simulink model "Simu_2"  (R2024a)
settings: Solver=VariableStepAuto  StartTime=0.0  StopTime=10  FixedStep=1e-4  RelTol=1e-3
undefined symbols (not defined in the file): B, K, kd, ki, kp, M, T
libraries: dspsrcs4 x2, slpidlib x1
settings Model: Creator=a2152355  LastModifiedBy=a2152355

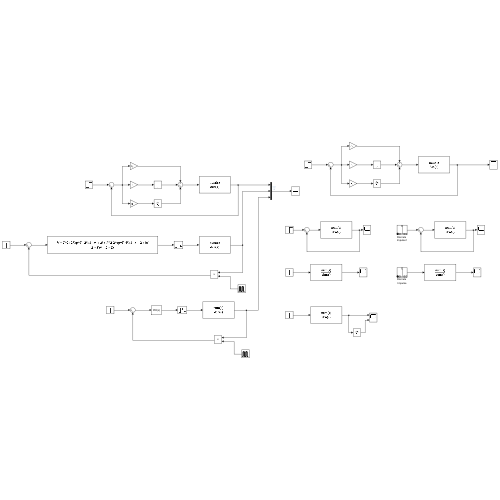
[thumbnail: Simulink's stored preview of the top-level diagram]
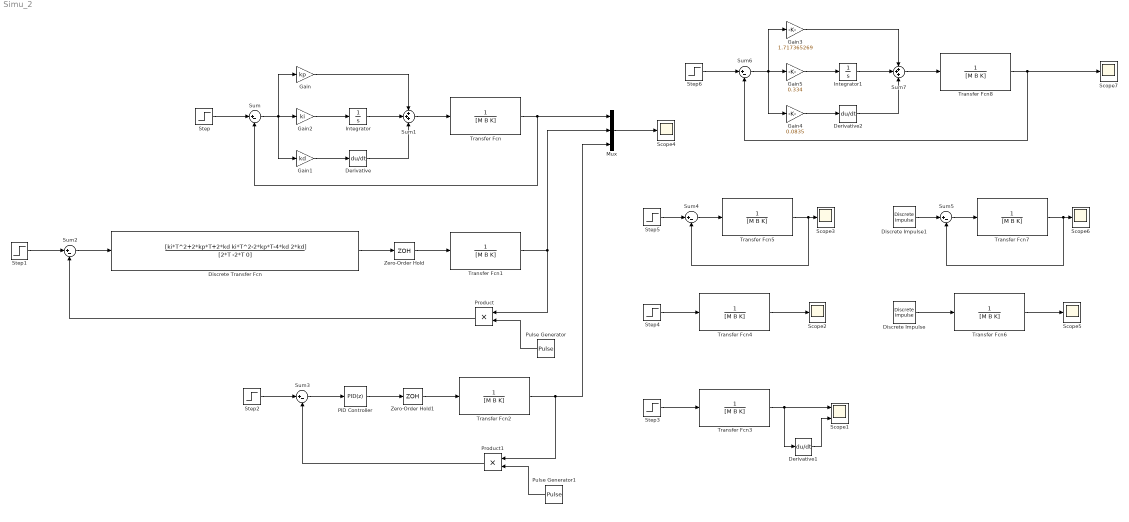
== system Simu_2 ==
  Derivative : Derivative
  Derivative1 : Derivative
  Derivative2 : Derivative
  Discrete Transfer Fcn : DiscreteTransferFcn  Numerator=[ki*T^2+2*kp*T+2*kd ki*T^2-2*kp*T-4*kd 2*kd]  Denominator=[2*T -2*T 0]
  Discrete Impulse : dspsrcs4/Discrete  Impulse  Delay=0  SampleTime=1  FrameSample=1  OutputFrames=off  dataType=double  isSigned=on  wordLen=16  udDataType=sfix(16)  fracBitsMode=Best precision  numFracBits=15  OutDataTypeStr=double  LastOutDataTypeStr=double
  Discrete Impulse1 : dspsrcs4/Discrete  Impulse  Delay=0  SampleTime=1  FrameSample=1  OutputFrames=off  dataType=double  isSigned=on  wordLen=16  udDataType=sfix(16)  fracBitsMode=Best precision  numFracBits=15  OutDataTypeStr=double  LastOutDataTypeStr=double
  Gain : Gain  Gain=kp
  Gain1 : Gain  Gain=kd
  Gain2 : Gain  Gain=ki
  Gain3 : Gain  Gain=1.717365269
  Gain4 : Gain  Gain=0.0835
  Gain5 : Gain  Gain=0.334
  Integrator : Integrator
  Integrator1 : Integrator
  Mux : Mux  Inputs=3
  PID Controller : slpidlib/PID Controller  Controller=PID  Form=Parallel  TimeDomain=Discrete-time  UseExternalTs=off  SampleTime=T  IntegratorMethod=Forward Euler  FilterMethod=Forward Euler  ControllerParametersSource=internal  P=kp  I=ki  UseKiTs=off  D=kd  UseExternalDerivativeSource=off  N=100  UseFilter=on  TunerSelectOption=Transfer Function Based (PID Tuner App)  InitialConditionSource=internal  InitialConditionForIntegrator=0  InitialConditionForFilter=0  DifferentiatorICPrevScaledInput=0  ExternalReset=none  TrackingMode=off  Kt=1  LimitOutput=off  SatLimitsSource=internal  UpperSaturationLimit=inf  LowerSaturationLimit=-inf  LinearizeAsGain=on  AntiWindupMode=none  Kb=1  LimitIntegrator=off  UpperIntegratorSaturationLimit=inf  LowerIntegratorSaturationLimit=-inf  POutMin=[]  POutMax=[]  IOutMin=[]  IOutMax=[]  DOutMin=[]  DOutMax=[]  NOutMin=[]  NOutMax=[]  SumOutMin=[]  SumOutMax=[]  SaturationOutMin=[]  SaturationOutMax=[]  PParamMin=[]  PParamMax=[]  IParamMin=[]  IParamMax=[]  DParamMin=[]  DParamMax=[]  NParamMin=[]  NParamMax=[]  KbParamMin=[]  KbParamMax=[]  KtParamMin=[]  KtParamMax=[]  KbOutMin=[]  KbOutMax=[]  KtOutMin=[]  KtOutMax=[]  IntegratorOutMin=[]  IntegratorOutMax=[]  FilterOutMin=[]  FilterOutMax=[]  SumI1OutMin=[]  SumI1OutMax=[]  SumI2OutMin=[]  SumI2OutMax=[]  SumI3OutMin=[]  SumI3OutMax=[]  SumI4OutMin=[]  SumI4OutMax=[]  SumDOutMin=[]  SumDOutMax=[]  DifferentiatorOutMin=[]  DifferentiatorOutMax=[]  FilterDiffOutCoefMin=[]  FilterDiffOutCoefMax=[]  ReciprocalOutMin=[]  ReciprocalOutMax=[]  SumDenOutMin=[]  SumDenOutMax=[]  SumNumOutMin=[]  SumNumOutMax=[]  DivideOutMin=[]  DivideOutMax=[]  UdiffTsProdOutMin=[]  UdiffTsProdOutMax=[]  NTsProdOutMin=[]  NTsProdOutMax=[]  UintegralTsProdOutMin=[]  UintegralTsProdOutMax=[]  UngainTsProdOutMin=[]  UngainTsProdOutMax=[]  ClampingZeroOutDataTypeStr=Inherit: Inherit via back propagation  ClampingZeroOutMin=[]  ClampingZeroOutMax=[]  FilterDenConstantOutDataTypeStr=Inherit: Inherit via back propagation  FilterDenConstantOutMin=[]  FilterDenConstantOutMax=[]  PCopyOutDataTypeStr=Inherit: Inherit via back propagation  PCopyOutMin=[]  PCopyOutMax=[]  NCopyOutDataTypeStr=Inherit: Inherit via back propagation  NCopyOutMin=[]  NCopyOutMax=[]  IntegratorContinuousStateAttributes=''  IntegratorStateMustResolveToSignalObject=off  IntegratorRTWStateStorageClass=Auto  FilterContinuousStateAttributes=''  FilterStateMustResolveToSignalObject=off  FilterRTWStateStorageClass=Auto  ParallelPVariant=InternalParameters  IdealPVariant=Disabled  IVariant=InternalParameters  DVariant=InternalParameters  IntegratorVariant=Discrete  SatVariant=Disabled  AWVariant=Passthrough  PCopyVariant=Disabled  TRVariant=Disabled  FdbkBlocksVariant=Forward  IdealPFdbkVariant=Disabled  SatFdbkVariant=Disabled  DerivativeFilterVariant=ForwardEulerFilter  NVariant=InternalParameters  NCopyVariant=Disabled  FilterICVariant=InternalICsFilter  IntegratorICVariant=InternalICs  ExternalResetVariant=Disabled  TRSumVariant=Passthrough  SumFdbkVariant=Disabled  SumVariant=Sum_PID  TsampFilterVariant=InternalTs  TsampNgainVariant=Passthrough  TsampIntegralVariant=Disabled_SignalSpec  ExternalSaturationOutDataTypeStr=Inherit: Same as second input  DerivativeSourceVariant=ErrorSignal
  Product : Product
  Product1 : Product
  Pulse Generator : DiscretePulseGenerator  PulseType=Time based  Period=T  PulseWidth=0.1
  Pulse Generator1 : DiscretePulseGenerator  PulseType=Time based  Period=T  PulseWidth=0.1
  Scope1 : Scope  NumInputPorts=2
  Scope{2..7} (6 alike) : Scope
  Step{,1..6} (7 alike) : Step  SampleTime=0
  Sum{,2..6} (6 alike) : Sum  Inputs=|+-
  Sum1 : Sum  Inputs=+++
  Sum7 : Sum  Inputs=+++
  Transfer Fcn{,1..8} (9 alike) : TransferFcn  Denominator=[M B K]
  Zero-Order Hold : ZeroOrderHold  SampleTime=T
  Zero-Order Hold1 : ZeroOrderHold  SampleTime=T
  wires:
  Transfer Fcn/1 -> Mux/1, Sum/2
  Sum/1 -> Gain2/1, Gain/1, Gain1/1
  Step/1 -> Sum/1
  Gain1/1 -> Derivative/1
  Derivative/1 -> Sum1/3
  Integrator/1 -> Sum1/2
  Gain/1 -> Sum1/1
  Gain2/1 -> Integrator/1
  Sum1/1 -> Transfer Fcn/1
  Transfer Fcn1/1 -> Product/1, Mux/2
  Pulse Generator/1 -> Product/2
  Zero-Order Hold/1 -> Transfer Fcn1/1
  Discrete Transfer Fcn/1 -> Zero-Order Hold/1
  Product/1 -> Sum2/2
  Sum2/1 -> Discrete Transfer Fcn/1
  Step1/1 -> Sum2/1
  Zero-Order Hold1/1 -> Transfer Fcn2/1
  Product1/1 -> Sum3/2
  Transfer Fcn2/1 -> Product1/1, Mux/3
  Pulse Generator1/1 -> Product1/2
  Step2/1 -> Sum3/1
  Sum3/1 -> PID Controller/1
  PID Controller/1 -> Zero-Order Hold1/1
  Step3/1 -> Transfer Fcn3/1
  Transfer Fcn3/1 -> Derivative1/1, Scope1/1
  Derivative1/1 -> Scope1/2
  Transfer Fcn4/1 -> Scope2/1
  Step4/1 -> Transfer Fcn4/1
  Transfer Fcn5/1 -> Scope3/1, Sum4/2
  Sum4/1 -> Transfer Fcn5/1
  Step5/1 -> Sum4/1
  Mux/1 -> Scope4/1
  Transfer Fcn6/1 -> Scope5/1
  Discrete Impulse/1 -> Transfer Fcn6/1
  Discrete Impulse1/1 -> Sum5/1
  Sum5/1 -> Transfer Fcn7/1
  Transfer Fcn7/1 -> Scope6/1, Sum5/2
  Derivative2/1 -> Sum7/3
  Gain3/1 -> Sum7/1
  Integrator1/1 -> Sum7/2
  Gain5/1 -> Integrator1/1
  Step6/1 -> Sum6/1
  Sum7/1 -> Transfer Fcn8/1
  Gain4/1 -> Derivative2/1
  Sum6/1 -> Gain5/1, Gain3/1, Gain4/1
  Transfer Fcn8/1 -> Scope7/1, Sum6/2
